simulink model "Simulink_drone_BF_final"  (R2025b)
settings: Solver=VariableStepAuto  StartTime=0.0  StopTime=10.0  RelTol=1e-3
undefined symbols (not defined in the file): A, B, bool, C, D, dt_realtime, init, K, K_default, Ki, params, pert, x_init
libraries: cstblocks x3, simulink x3, uavsim3dlib x1, sim3dlib x1, aerolibanimutils x1
settings Model: Creator=guilb  LastModifiedBy=pierr

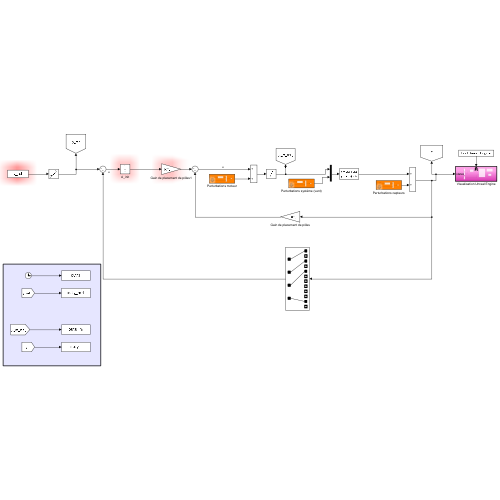
[thumbnail: Simulink's stored preview of the top-level diagram]
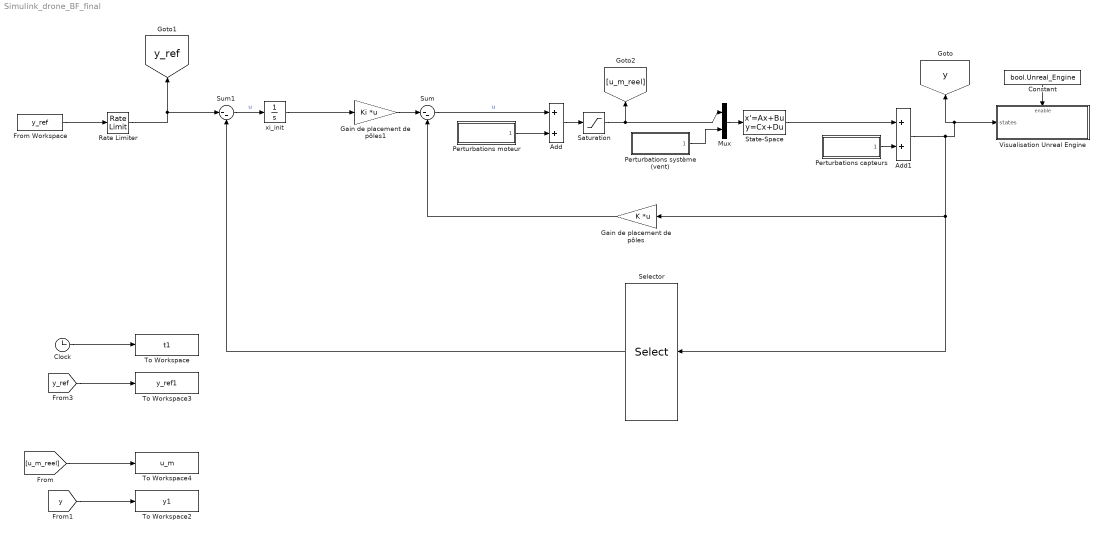
== system Simulink_drone_BF_final ==
  Add : Sum
  Add1 : Sum
  Clock : Clock
  Constant : Constant  Value=bool.Unreal_Engine
  From Workspace : FromWorkspace  VariableName=y_ref
  Gain de placement de pôles : Gain  Gain=K  Multiplication=Matrix(K*u)
  Gain de placement de pôles1 : Gain  Gain=Ki  Multiplication=Matrix(K*u)
  Mux : Mux  Inputs=2
  Perturbations capteurs : Subsystem  mask{perturbation=pert.capteur, Ts=dt_realtime}
      mask prompts: perturbation "modèle de perturbation"; Ts "echantillonage"
      mask DialogControl ParameterGroupVar Prompt: Configuration - bruit blanc filtré
  Perturbations moteur : Subsystem  mask{perturbation=pert.motor, Ts=dt_realtime}
      mask prompts: perturbation "modèle de perturbation"; Ts "echantillonage"
      mask DialogControl ParameterGroupVar Prompt: Configuration - bruit blanc filtré
  Perturbations système (vent) : Subsystem  mask{perturbation=pert.vent, Ts=dt_realtime}
      mask prompts: perturbation "modèle de perturbation"; Ts "echantillonage"
      mask DialogControl ParameterGroupVar Prompt: Configuration - bruit blanc filtré
  Rate Limiter : RateLimiter  RisingSlewLimit=params.v_ref  FallingSlewLimit=-params.v_ref  SampleTimeMode=inherited  InitialCondition=init([1 3 5 11])
  Saturation : Saturate  UpperLimit=params.Wmot2_sat  LowerLimit=-params.Wmot2_sat
  Selector : Selector  InputPortWidth=12  IndexOptions=Index vector (dialog)  Indices=[1, 3, 5, 11]  OutputSizes=1
  State-Space : StateSpace  A=A  B=B  C=C  D=D  InitialCondition=0
  Sum : Sum  Inputs=|--
  Sum1 : Sum  Inputs=|--
  To Workspace : ToWorkspace  VariableName=t1  SaveFormat=Timeseries  SampleTime=-1
  To Workspace2 : ToWorkspace  VariableName=y1  SaveFormat=Timeseries  SampleTime=-1
  To Workspace3 : ToWorkspace  VariableName=y_ref1  SaveFormat=Timeseries  SampleTime=-1
  To Workspace4 : ToWorkspace  VariableName=u_m  SaveFormat=Timeseries  SampleTime=-1
  Visualisation Unreal Engine : Subsystem
  xi_init : Integrator  InitialCondition=-pinv(Ki)*K_default*init(1:12)
  tag scope: y=global, y_ref=global
  wires:
  Constant/1 -> Visualisation Unreal Engine/Enable
  From Workspace/1 -> Rate Limiter/1
  Gain de placement de pôles/1 -> Sum/2
  Gain de placement de pôles1/1 -> Sum/1
  Saturation/1 -> [u_m_reel], Mux/1
  [y_ref] -> To Workspace3/1
  [y] -> To Workspace2/1
  Clock/1 -> To Workspace/1
  [u_m_reel] -> To Workspace4/1
  Rate Limiter/1 -> Sum1/1, [y_ref]
  Perturbations moteur/1("  ") -> Add/2
  Add/1 -> Saturation/1
  Sum/1 -> Add/1  "u"
  Mux/1 -> State-Space/1
  Perturbations système (vent)/1("  ") -> Mux/2
  Perturbations capteurs/1("  ") -> Add1/2
  State-Space/1 -> Add1/1
  Add1/1 -> Selector/1, Gain de placement de pôles/1, Visualisation Unreal Engine/1(states), [y]
  xi_init/1 -> Gain de placement de pôles1/1
  Sum1/1 -> xi_init/1  "u"
  Selector/1 -> Sum1/2

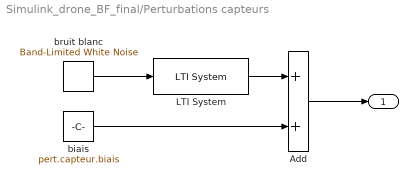
== system Simulink_drone_BF_final/Perturbations capteurs ==
  Add : Sum
  LTI System : cstblocks/LTI System  sys=pert.capteur.filtre  IC=[]  PadeOrder=0
  biais : Constant  Value=pert.capteur.biais  SampleTime=Ts
  bruit blanc : simulink/Sources/Band-Limited White Noise  Cov=pert.capteur.noise_power  Ts=Ts  seed=pert.capteur.seed
  "  " : Outport
  wires:
  Add/1 -> "  "/1
  biais/1 -> Add/2
  LTI System/1 -> Add/1
  bruit blanc/1 -> LTI System/1

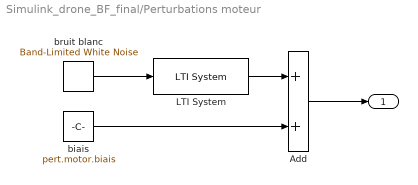
== system Simulink_drone_BF_final/Perturbations moteur ==
  Add : Sum
  LTI System : cstblocks/LTI System  sys=pert.motor.filtre  IC=[]  PadeOrder=0
  biais : Constant  Value=pert.motor.biais  SampleTime=Ts
  bruit blanc : simulink/Sources/Band-Limited White Noise  Cov=pert.motor.noise_power  Ts=Ts  seed=pert.motor.seed
  "  " : Outport
  wires:
  Add/1 -> "  "/1
  biais/1 -> Add/2
  LTI System/1 -> Add/1
  bruit blanc/1 -> LTI System/1

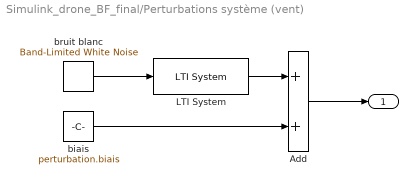
== system Simulink_drone_BF_final/Perturbations système (vent) ==
  Add : Sum
  LTI System : cstblocks/LTI System  sys=pert.vent.filtre  IC=[]  PadeOrder=0
  biais : Constant  Value=perturbation.biais  SampleTime=Ts
  bruit blanc : simulink/Sources/Band-Limited White Noise  Cov=pert.vent.noise_power  Ts=Ts  seed=pert.vent.seed
  "  " : Outport
  wires:
  Add/1 -> "  "/1
  biais/1 -> Add/2
  LTI System/1 -> Add/1
  bruit blanc/1 -> LTI System/1

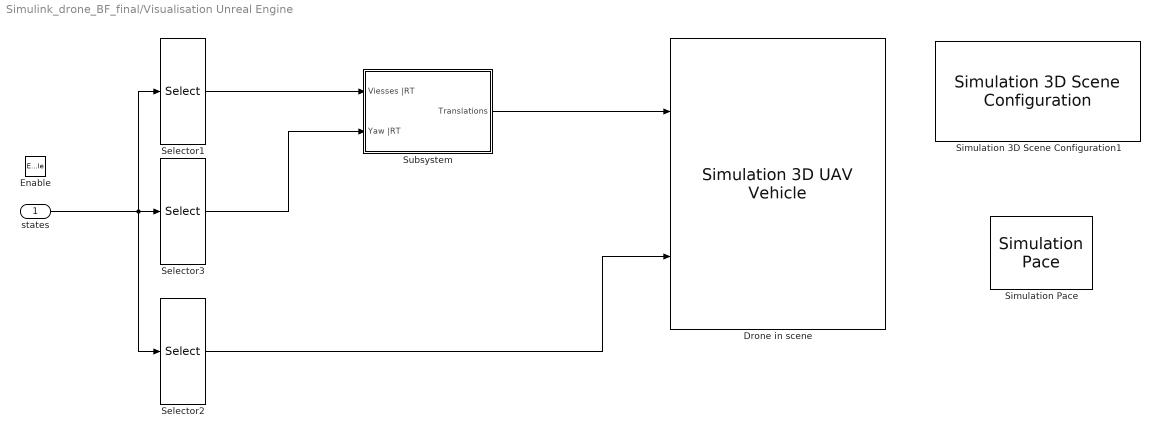
== system Simulink_drone_BF_final/Visualisation Unreal Engine ==
  states : Inport
  Enable : EnablePort
  Drone in scene : uavsim3dlib/Simulation 3D UAV Vehicle  Priority=-1  Mesh=Quadrotor  MeshPath=/MathWorksUAVContent/UAVs/HexaRotorUAV/HexaRotor.HexaRotor  Color=Black  ActorName=Razmo  UseGlobalFrame=off  InitialTranslation=[0 0 0]  InitialRotation=[0 0 0]  InitialTranslationGlobal=[0 0 0]  InitialGeoOrigin=[0 0 0]  InitialRotationGlobal=[0 0 0]  SampleTime=-1  ActorType=SimulinkVehicle  ID=C  aMode=4  ActorTag=Razmo
  Selector1 : Selector  InputPortWidth=12  IndexOptions=Index vector (dialog)  Indices=[2 4 6]  OutputSizes=1
  Selector2 : Selector  InputPortWidth=12  IndexOptions=Index vector (dialog)  Indices=[11 9 7]  OutputSizes=1
  Selector3 : Selector  InputPortWidth=12  IndexOptions=Index vector (dialog)  Indices=11  OutputSizes=1
  Simulation 3D Scene Configuration1 : sim3dlib/Simulation 3D Scene Configuration  Priority=0  ProjectFormat=Default Scenes  SceneDesc=US city block  ProjectName=C:\Program Files\MATLAB\R2025b\toolbox\shared\sim3d_projects\automotive_project_windows\UE\WindowsNoEditor\VehicleSimulation.exe  ScenePath=/Game/Maps/USCityBlock  EnableOpenDRIVE=off  vehTagList={'Custom';'Razmo';'Scene Origin'}  vehTag=Razmo  AttachedCameraRelativeTranslation=[0 0 0]  FreeCameraDefaultInitialTranslation=[-6, 0, 2]  AttachedCameraRelativeRotation=[0 0 0]  FreeCameraDefaultInitialRotation=[0, -15, 0]  ViewpointName=Razmo  FreeCameraInitialTranslation=[0 0 0]  ViewpointTranslation=[0 0 0]  FreeCameraInitialRotation=[0 0 0]  ViewpointRotation=[0 0 0]  OpVisEn=off  Ts=dt_realtime  EnableWindow=on  EnableRemoteAccess=off  EnableWeather=off  SunAzimuth=90  SunAltitude=40.0  EnableGeospatialSun=off  Latitude=0  Longitude=0  Date=2023-01-01  Time=10:30:00  GeoTimeZone=-5.0  SunDaylightSaving=off  wind=1  clouds=10  EnableVolumetricClouds=off  CloudCoverage=0  CloudAltitude=6  fog=0  rain=0  RaindropsEffect=off  SnowDensity=0  EnableGeospatial=off  TilesetSource=Earth terrain  UseTrueOrigin=off  OriginHeight=200  OriginLatitude=40.744652  OriginLongitude=-73.988864  MapStyle=Aerial  AdditionalAssetIDs=[]  UseAdvancedSunSky=off  SolarTime=11  TimeZone=-5  Day=21  Month=9  Year=2022  UseDaylightSavingTime=on  DSTStartDay=10  DSTStartMonth=3  DSTEndDay=3  DSTEndMonth=11  DSTSwitchHour=2  sensorTag=MainCamera1  sensorId=1  sensorName=MainCamera1  mountLoc=Origin  offsetFlag=off  tmountOffset=[0, 0, 0]  rmountOffset=[0, 0, 0]  HorizontalResolution=1280  VerticalResolution=720  HorizontalFOV=60  mountPoint=[0 0 0]  mountOrientation=[0 0 0]  aMode=4  ID=1  GeoTrigger=Inactive  ViewNameList={'Custom', 'Razmo'}  ViewTranslationList={'[0 0 0]', '[0 0 0]'}  ViewRotationList={'[0 0 0]', '[0 0 0]'}
      settings: LibrarySourceBlock=uavsim3dlib/Simulation 3D Scene Configuration
  Simulation Pace : aerolibanimutils/Simulation Pace  SimulationPace=1  SleepMode=Auto  OutputPaceError=off  SampleTime=dt_realtime
  Subsystem : Subsystem
  wires:
  states/1 -> Selector1/1, Selector2/1, Selector3/1
  Selector2/1 -> Drone in scene/2
  Selector1/1 -> Subsystem/1(Viesses |RT)
  Selector3/1 -> Subsystem/2("Yaw |RT ")
  Subsystem/1(Translations) -> Drone in scene/1

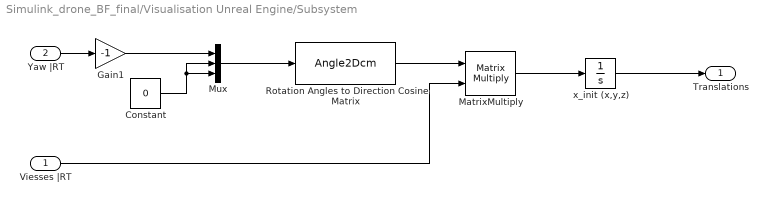
== system Simulink_drone_BF_final/Visualisation Unreal Engine/Subsystem ==
  Viesses |RT : Inport
  "Yaw |RT " : Inport  Port=2
  Constant : Constant  Value=0
  Gain1 : Gain  Gain=-1
  MatrixMultiply : Product  Multiplication=Matrix(*)
  Mux : Mux  Inputs=3
  Rotation Angles to Direction Cosine Matrix : Angle2Dcm
      settings: AttributesFormatString=Rotation Order: %<rotationOrder>
  x_init (x,y,z) : Integrator  InitialCondition=[x_init(1) ; x_init(3) ; x_init(5)]
  Translations : Outport
  wires:
  Constant/1 -> Mux/2, Mux/3
  x_init (x,y,z)/1 -> Translations/1
  MatrixMultiply/1 -> x_init (x,y,z)/1
  Mux/1 -> Rotation Angles to Direction Cosine Matrix/1
  Rotation Angles to Direction Cosine Matrix/1 -> MatrixMultiply/1
  "Yaw |RT "/1 -> Gain1/1
  Viesses |RT/1 -> MatrixMultiply/2
  Gain1/1 -> Mux/1
